simulink model "SpeedController"  (R2018a)
settings: Solver=VariableStepAuto  StartTime=0.0  StopTime=tf  RelTol=1e-6
values from neighbouring files (symbols this model uses):
  A = pi*2^2    (= 12.5663706144)    [TestSpeedController.m]
  atmo_height = 100000    [TestSpeedController.m]
  Cd = 0.75    [TestSpeedController.m]
  g0 = abs(Grav(physparams.earthradius_m,physparams.earthgrav,1.0))    [RocketDynamicsIGM.m]    (also in TestPropTraj.m = -1*Grav(R0,physparams.earthgrav,1.0); TestSpeedController.m = 9.81; testIGM.m = -1*Grav(R0,physparams.earthgrav,1.0))
  Isp = 50000    [TestSpeedController.m]
  Kd = 0    [TestSpeedController.m]
  Ki = 500    [TestSpeedController.m]
  Kp = 1000    [TestSpeedController.m]
  m0 = 8000    [TestSpeedController.m]
  mu_earth = 3.98600441*10^14    (= 398600441000000)    [TestSpeedController.m]
  radius_earth = 6731000    [TestSpeedController.m]
  Tmax = 5*g0*m0    (= 392400)    [TestSpeedController.m]
  Tmin = 0.5*g0*m0    (= 39240)    [TestSpeedController.m]
libraries: simulink x1
settings Model: Creator=corey  LastModifiedBy=corey

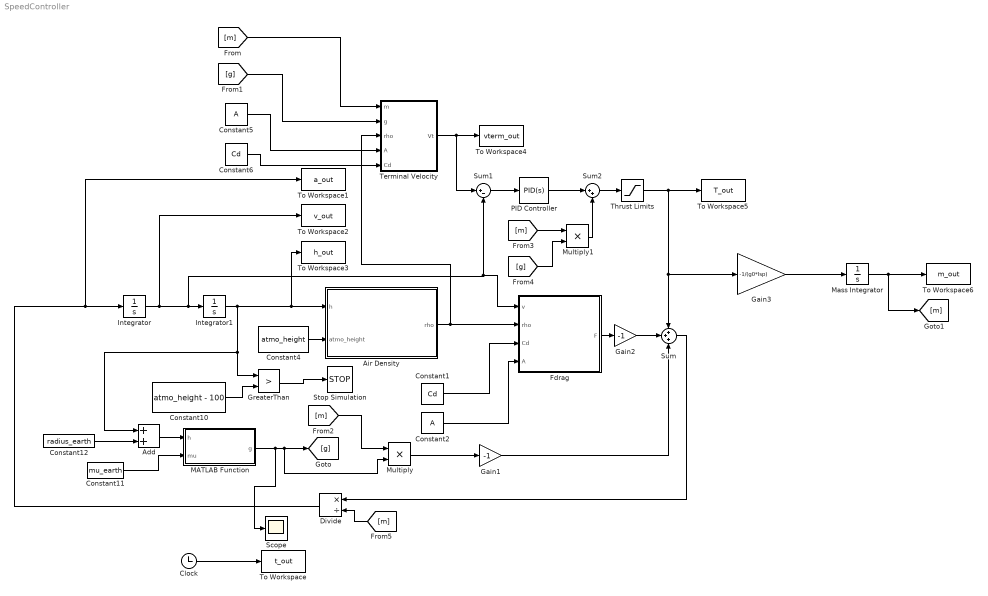
== system SpeedController ==
  Add : Sum
  Air Density : MATLAB Function  TreatAsAtomicUnit=on
  Clock : Clock
  Constant1 : Constant  Value=Cd
  Constant10 : Constant  Value=atmo_height - 100
  Constant11 : Constant  Value=mu_earth
  Constant12 : Constant  Value=radius_earth
  Constant2 : Constant  Value=A
  Constant4 : Constant  Value=atmo_height
  Constant5 : Constant  Value=A
  Constant6 : Constant  Value=Cd
  Divide : Product  Inputs=*/
  Fdrag : MATLAB Function  TreatAsAtomicUnit=on
  Gain1 : Gain  Gain=-1
  Gain2 : Gain  Gain=-1
  Gain3 : Gain  Gain=-1/(g0*Isp)
  GreaterThan : RelationalOperator  Operator=>  OutDataTypeStr=boolean  RndMeth=Simplest
  Integrator : Integrator
  Integrator1 : Integrator
  MATLAB Function : MATLAB Function  TreatAsAtomicUnit=on
  Mass Integrator : Integrator  InitialCondition=m0
  Multiply : Product
  Multiply1 : Product
  PID Controller : simulink/Continuous/PID Controller  Controller=PID  TimeDomain=Continuous-time  SampleTime=-1  IntegratorMethod=Forward Euler  FilterMethod=Forward Euler  Form=Parallel  UseFilter=on  ControllerParametersSource=internal  P=Kp  I=Ki  D=Kd  N=100  InitialConditionSource=internal  InitialConditionForIntegrator=0  InitialConditionForFilter=0  ExternalReset=none  LimitOutput=off  UpperSaturationLimit=inf  LowerSaturationLimit=-inf  LinearizeAsGain=on  AntiWindupMode=none  Kb=1  TrackingMode=off  Kt=1  PParamMin=[]  PParamMax=[]  IParamMin=[]  IParamMax=[]  DParamMin=[]  DParamMax=[]  NParamMin=[]  NParamMax=[]  KbParamMin=[]  KbParamMax=[]  KtParamMin=[]  KtParamMax=[]  POutMin=[]  POutMax=[]  IOutMin=[]  IOutMax=[]  DOutMin=[]  DOutMax=[]  NOutMin=[]  NOutMax=[]  KbOutMin=[]  KbOutMax=[]  KtOutMin=[]  KtOutMax=[]  IntegratorOutMin=[]  IntegratorOutMax=[]  FilterOutMin=[]  FilterOutMax=[]  SumOutMin=[]  SumOutMax=[]  SumI1OutMin=[]  SumI1OutMax=[]  SumI2OutMin=[]  SumI2OutMax=[]  SumI3OutMin=[]  SumI3OutMax=[]  SumDOutMin=[]  SumDOutMax=[]  SaturationOutMin=[]  SaturationOutMax=[]  IntegratorContinuousStateAttributes=''  IntegratorStateMustResolveToSignalObject=off  IntegratorRTWStateStorageClass=Auto  FilterContinuousStateAttributes=''  FilterStateMustResolveToSignalObject=off  FilterRTWStateStorageClass=Auto  DifferentiatorICPrevScaledInput=0  DifferentiatorOutMin=[]  DifferentiatorOutMax=[]  FilterDiffOutCoefMin=[]  FilterDiffOutCoefMax=[]  SumDenOutMin=[]  SumDenOutMax=[]  SumNumOutMin=[]  SumNumOutMax=[]  ReciprocalOutMin=[]  ReciprocalOutMax=[]  DivideOutMin=[]  DivideOutMax=[]  TunerSelectOption=Transfer Function Based (PID Tuner App)
  Scope : Scope
  Stop Simulation : Stop
  Sum : Sum  Inputs=+++
  Sum1 : Sum  Inputs=|+-
  Sum2 : Sum  Inputs=|++
  Terminal Velocity : MATLAB Function  TreatAsAtomicUnit=on
  Thrust Limits : Saturate  UpperLimit=Tmax  LowerLimit=Tmin
  To Workspace : ToWorkspace  VariableName=t_out  SampleTime=-1
  To Workspace1 : ToWorkspace  VariableName=a_out  SampleTime=-1
  To Workspace2 : ToWorkspace  VariableName=v_out  SampleTime=-1
  To Workspace3 : ToWorkspace  VariableName=h_out  SampleTime=-1
  To Workspace4 : ToWorkspace  VariableName=vterm_out  SampleTime=-1
  To Workspace5 : ToWorkspace  VariableName=T_out  SampleTime=-1
  To Workspace6 : ToWorkspace  VariableName=m_out  SampleTime=-1
  wires:
  Integrator/1 -> To Workspace2/1, Fdrag/1(v), Sum1/2, Integrator1/1
  Integrator1/1 -> To Workspace3/1, Air Density/1(h), Add/1, GreaterThan/1
  Constant4/1 -> Air Density/2(atmo_height)
  Air Density/1(rho) -> Fdrag/2(rho), Terminal Velocity/3(rho)
  Constant1/1 -> Fdrag/3(Cd)
  Constant2/1 -> Fdrag/4(A)
  Fdrag/1(F) -> Gain2/1
  Sum/1 -> Divide/1
  Divide/1 -> To Workspace1/1, Integrator/1
  Multiply/1 -> Gain1/1
  Terminal Velocity/1(Vt) -> To Workspace4/1, Sum1/1
  Sum1/1 -> PID Controller/1
  Clock/1 -> To Workspace/1
  Constant5/1 -> Terminal Velocity/4(A)
  Constant6/1 -> Terminal Velocity/5(Cd)
  MATLAB Function/1(g) -> Scope/1, Multiply/2, [g]
  Gain1/1 -> Sum/3
  [m] -> Multiply/1
  [m] -> Terminal Velocity/1(m)
  [g] -> Terminal Velocity/2(g)
  PID Controller/1 -> Sum2/1
  Sum2/1 -> Thrust Limits/1
  Multiply1/1 -> Sum2/2
  Thrust Limits/1 -> To Workspace5/1, Gain3/1, Sum/1
  Gain2/1 -> Sum/2
  GreaterThan/1 -> Stop Simulation/1
  Constant10/1 -> GreaterThan/2
  Gain3/1 -> Mass Integrator/1
  Mass Integrator/1 -> [m], To Workspace6/1
  Constant11/1 -> MATLAB Function/2(mu)
  Add/1 -> MATLAB Function/1(h)
  Constant12/1 -> Add/2
  [m] -> Multiply1/1
  [g] -> Multiply1/2
  [m] -> Divide/2

== matlab function SpeedController/Fdrag ==
  data: v input; F output; rho input; Cd input; A input
function F = DragBlock(v, rho, Cd, A)

%vectorize velocity
v_vec = [v; 0];

%produces a 2-D drag
Fdrag = Drag(v_vec, rho, Cd, A);

%get scalar drag
F = norm(Fdrag);

== matlab function SpeedController/Air Density ==
  data: h input; rho output; atmo_height input
function rho = AirDensityBlock(h,atmo_height)

rho = AirDensity(h, atmo_height);

== matlab function SpeedController/Terminal Velocity ==
  data: m input; Vt output; g input; rho input; A input; Cd input
function Vt = TermVel(m,g,rho,A,Cd)

Vt = sqrt((2*m*g)/(rho*A*Cd));

== matlab function SpeedController/MATLAB Function ==
  data: h input; g output; mu input
function g = GravAccel(h, mu)

%position
r = [h; 0];

%calculate gravity vector
g_vec = Grav(r, mu, 1);

g = norm(g_vec);
